simulink model "DUALportRAMinterface_v2"  (R2024a)
settings: Solver=FixedStepDiscrete  StartTime=0.0  StopTime=20  RelTol=1e-3
values from neighbouring files (symbols this model uses):
  Ts = 1/Fs    (= 7.50007500075e-06)    [new_generation_coeff.m]    (also in simon_test.m; simple_fft_test.m = 1/F; testPSD_c2d.m; testPSD_simulink.m)
undefined symbols (not defined in the file or in its folder): magnitude
libraries: hdlsllib x226, embmathops x6, simulink x1, hdlmdlgenlib x1, dsphdlxfrm2 x1
(part 2 of 5)

== system DUALportRAMinterface_v2/PL/integration_block1/FIFO_system1 ==
  data_in : Inport
  enable_output : Inport  Port=2  OutDataTypeStr=boolean
  load_fifo : Inport  Port=3  OutDataTypeStr=boolean
  Add1 : Sum  OutDataTypeStr=fixdt(0,13,0)
  Chart1 : Stateflow chart  TreatAsAtomicUnit=on
      settings: PortSchema="{\"entries\":[{\"content\":{\"sides\":[{\"content\":{\"connectorIds\":[\"In2\"]},\"type\":\"ConnectorPlacement.EquallySpacedRectSide\",\"uuid\":\"9d6f18ef-7bce-40b0-94a2-758e33355834\"},{\"content\":{\"connectorIds\":[\"Out1\"],\"side\":\"RIGHT\"},\"type\":\"ConnectorPlacement.EquallySpacedRectSide\",\"uuid\":\"7bab70ba-8111-4145-9c29-33f98ce79820\"},{\"content\":{\"side\":\"TOP\"},\"type\":\"ConnectorPlacement.EquallySpacedRectSide\",\"uuid\":\"d3288235-814f-4c71-bec2-04d07c53d63c\"},{\"content\":{\"connectorIds\":[\"In1\"],\"side\":\"BOTTOM\"},\"type\":\"ConnectorPlacement.EquallySpacedRectSide\",\"uuid\":\"018953e5-55f4-4114-8f5d-132f3f7565f7\"}]},\"type\":\"ConnectorPlacement.EquallySpacedConnector\",\"uuid\":\"70011da9-c6ae-4e69-953f-1d8cbe8c7c12\"}],\"packageUris\":[\"http://schema.mathworks.com/mf0/Connector/R2020b\"],\"version\":\"1.0\"}"
  Chart2 : Stateflow chart  TreatAsAtomicUnit=on
      settings: PortSchema="{\"entries\":[{\"content\":{\"sides\":[{\"content\":{\"connectorIds\":[\"In1\"]},\"type\":\"ConnectorPlacement.EquallySpacedRectSide\",\"uuid\":\"9d6f18ef-7bce-40b0-94a2-758e33355834\"},{\"content\":{\"connectorIds\":[\"Out1\"],\"side\":\"RIGHT\"},\"type\":\"ConnectorPlacement.EquallySpacedRectSide\",\"uuid\":\"7bab70ba-8111-4145-9c29-33f98ce79820\"},{\"content\":{\"connectorIds\":[\"In2\"],\"side\":\"TOP\"},\"type\":\"ConnectorPlacement.EquallySpacedRectSide\",\"uuid\":\"d3288235-814f-4c71-bec2-04d07c53d63c\"}]},\"type\":\"ConnectorPlacement.EquallySpacedConnector\",\"uuid\":\"70011da9-c6ae-4e69-953f-1d8cbe8c7c12\"}],\"packageUris\":[\"http://schema.mathworks.com/mf0/Connector/R2020b\"],\"version\":\"1.0\"}"
  Chart3 : Stateflow chart  TreatAsAtomicUnit=on
  Constant3 : Constant  OutDataTypeStr=fixdt(0,12,0)  SampleTime=Ts
  Constant4 : Constant  Value=0  OutDataTypeStr=fixdt(1,13,0)  SampleTime=Ts
  Delay : Delay  DelayLength=2048  InitialCondition=0  UseCircularBuffer=on
  Delay1 : Delay  DelayLength=1  InitialCondition=0  SampleTime=Ts
  Delay2 : Delay  DelayLength=1  InitialCondition=0  SampleTime=Ts
  Delay3 : Delay  DelayLength=1  InitialCondition=0
  HDL FIFO1 : hdlsllib/HDL RAMs/HDL FIFO  fifo_size=4096+2048+1  mode=Classic  ratio=1  push_msg=Warning  pop_msg=Warning  show_empty=off  show_full=on  show_num=off  LabelModeActiveChoice_Mode=Classic  rst_port=off
  Logical Operator : Logic  Operator=OR  IconShape=distinctive  AllPortsSameDT=off  OutDataTypeStr=boolean
  Logical Operator1 : Logic  IconShape=distinctive  AllPortsSameDT=off  OutDataTypeStr=boolean
  Logical Operator2 : Logic  IconShape=distinctive  AllPortsSameDT=off  OutDataTypeStr=boolean
  Logical Operator3 : Logic  Operator=XOR  IconShape=distinctive  AllPortsSameDT=off  OutDataTypeStr=boolean
  Logical Operator4 : Logic  IconShape=distinctive  AllPortsSameDT=off  OutDataTypeStr=boolean
  Logical Operator5 : Logic  Operator=XOR  IconShape=distinctive  AllPortsSameDT=off  OutDataTypeStr=boolean
  Logical Operator6 : Logic  Operator=XOR  IconShape=distinctive  AllPortsSameDT=off  OutDataTypeStr=boolean
  Switch1 : Switch  Criteria=u2 ~= 0  OutDataTypeStr=fixdt(0,13,0)  SaturateOnIntegerOverflow=off  InputSameDT=off
  Switch3 : Switch  Criteria=u2 ~= 0  SaturateOnIntegerOverflow=off  InputSameDT=off  OutDataTypeStr=Inherit: Same as first input
  tuneback : Delay  DelayLength=2048+4096+0  InitialCondition=0  UseCircularBuffer=on
  data_out : Outport
  data_valid : Outport  Port=2
  reset_fft : Outport  Port=3
  FIFO_full : Outport  Port=4
  wires:
  Delay1/1 -> Chart1/1(counter), Add1/1
  Logical Operator/1 -> HDL FIFO1/2
  HDL FIFO1/1 -> Switch3/3, data_out/1
  Switch1/1 -> Chart3/1(counter), Delay1/1
  Delay2/1 -> Logical Operator1/2
  enable_output/1 -> Chart1/2(en_out)
  Add1/1 -> Switch1/1
  Constant3/1 -> Add1/2
  HDL FIFO1/2 -> Delay3/1, Logical Operator6/1, Chart2/2(full)
  Switch3/1 -> HDL FIFO1/1
  Constant4/1 -> Switch1/3
  load_fifo/1 -> Chart2/1(load_FIFO1)
  data_in/1 -> Switch3/1
  Chart3/1(enable_pop) -> HDL FIFO1/3, Logical Operator1/1, Delay2/1, Logical Operator/2
  Chart1/1(enable_counter) -> Switch1/2
  Chart2/1(enable_push) -> Switch3/2, Logical Operator/1
  Delay/1 -> Logical Operator2/2
  Logical Operator2/1 -> Logical Operator3/1, Logical Operator5/1
  Logical Operator1/1 -> Logical Operator4/1, Logical Operator3/2, Logical Operator2/1, tuneback/1, Delay/1
  Logical Operator3/1 -> reset_fft/1
  tuneback/1 -> Logical Operator4/2
  Logical Operator4/1 -> Logical Operator5/2
  Logical Operator5/1 -> data_valid/1
  Logical Operator6/1 -> FIFO_full/1
  Delay3/1 -> Logical Operator6/2

== system DUALportRAMinterface_v2/PL/integration_block1/FIFO_system3 ==
  data_in : Inport
  enable_output : Inport  Port=2  OutDataTypeStr=boolean
  load_fifo : Inport  Port=3  OutDataTypeStr=boolean
  Add1 : Sum  OutDataTypeStr=fixdt(0,13,0)
  Chart1 : Stateflow chart  TreatAsAtomicUnit=on
      settings: PortSchema="{\"entries\":[{\"content\":{\"sides\":[{\"content\":{\"connectorIds\":[\"In2\"]},\"type\":\"ConnectorPlacement.EquallySpacedRectSide\",\"uuid\":\"9d6f18ef-7bce-40b0-94a2-758e33355834\"},{\"content\":{\"connectorIds\":[\"Out1\"],\"side\":\"RIGHT\"},\"type\":\"ConnectorPlacement.EquallySpacedRectSide\",\"uuid\":\"7bab70ba-8111-4145-9c29-33f98ce79820\"},{\"content\":{\"side\":\"TOP\"},\"type\":\"ConnectorPlacement.EquallySpacedRectSide\",\"uuid\":\"d3288235-814f-4c71-bec2-04d07c53d63c\"},{\"content\":{\"connectorIds\":[\"In1\"],\"side\":\"BOTTOM\"},\"type\":\"ConnectorPlacement.EquallySpacedRectSide\",\"uuid\":\"018953e5-55f4-4114-8f5d-132f3f7565f7\"}]},\"type\":\"ConnectorPlacement.EquallySpacedConnector\",\"uuid\":\"70011da9-c6ae-4e69-953f-1d8cbe8c7c12\"}],\"packageUris\":[\"http://schema.mathworks.com/mf0/Connector/R2020b\"],\"version\":\"1.0\"}"
  Chart2 : Stateflow chart  TreatAsAtomicUnit=on
      settings: PortSchema="{\"entries\":[{\"content\":{\"sides\":[{\"content\":{\"connectorIds\":[\"In1\"]},\"type\":\"ConnectorPlacement.EquallySpacedRectSide\",\"uuid\":\"9d6f18ef-7bce-40b0-94a2-758e33355834\"},{\"content\":{\"connectorIds\":[\"Out1\"],\"side\":\"RIGHT\"},\"type\":\"ConnectorPlacement.EquallySpacedRectSide\",\"uuid\":\"7bab70ba-8111-4145-9c29-33f98ce79820\"},{\"content\":{\"connectorIds\":[\"In2\"],\"side\":\"TOP\"},\"type\":\"ConnectorPlacement.EquallySpacedRectSide\",\"uuid\":\"d3288235-814f-4c71-bec2-04d07c53d63c\"}]},\"type\":\"ConnectorPlacement.EquallySpacedConnector\",\"uuid\":\"70011da9-c6ae-4e69-953f-1d8cbe8c7c12\"}],\"packageUris\":[\"http://schema.mathworks.com/mf0/Connector/R2020b\"],\"version\":\"1.0\"}"
  Chart3 : Stateflow chart  TreatAsAtomicUnit=on
  Constant3 : Constant  OutDataTypeStr=fixdt(0,12,0)  SampleTime=Ts
  Constant4 : Constant  Value=0  OutDataTypeStr=fixdt(1,13,0)  SampleTime=Ts
  Delay : Delay  DelayLength=2048  InitialCondition=0  UseCircularBuffer=on
  Delay1 : Delay  DelayLength=1  InitialCondition=0  SampleTime=Ts
  Delay2 : Delay  DelayLength=1  InitialCondition=0  SampleTime=Ts
  Delay3 : Delay  DelayLength=1  InitialCondition=0
  HDL FIFO1 : hdlsllib/HDL RAMs/HDL FIFO  fifo_size=4096+2048+1  mode=Classic  ratio=1  push_msg=Warning  pop_msg=Warning  show_empty=off  show_full=on  show_num=off  LabelModeActiveChoice_Mode=Classic  rst_port=off
  Logical Operator : Logic  Operator=OR  IconShape=distinctive  AllPortsSameDT=off  OutDataTypeStr=boolean
  Logical Operator1 : Logic  IconShape=distinctive  AllPortsSameDT=off  OutDataTypeStr=boolean
  Logical Operator2 : Logic  IconShape=distinctive  AllPortsSameDT=off  OutDataTypeStr=boolean
  Logical Operator3 : Logic  Operator=XOR  IconShape=distinctive  AllPortsSameDT=off  OutDataTypeStr=boolean
  Logical Operator4 : Logic  IconShape=distinctive  AllPortsSameDT=off  OutDataTypeStr=boolean
  Logical Operator5 : Logic  Operator=XOR  IconShape=distinctive  AllPortsSameDT=off  OutDataTypeStr=boolean
  Logical Operator6 : Logic  Operator=XOR  IconShape=distinctive  AllPortsSameDT=off  OutDataTypeStr=boolean
  Switch1 : Switch  Criteria=u2 ~= 0  OutDataTypeStr=fixdt(0,13,0)  SaturateOnIntegerOverflow=off  InputSameDT=off
  Switch3 : Switch  Criteria=u2 ~= 0  SaturateOnIntegerOverflow=off  InputSameDT=off  OutDataTypeStr=Inherit: Same as first input
  tuneback : Delay  DelayLength=2048+4096+0  InitialCondition=0  UseCircularBuffer=on
  data_out : Outport
  data_valid : Outport  Port=2
  reset_fft : Outport  Port=3
  FIFO_full : Outport  Port=4
  wires:
  Delay3/1 -> Logical Operator6/2
  Logical Operator6/1 -> FIFO_full/1
  Logical Operator5/1 -> data_valid/1
  Logical Operator4/1 -> Logical Operator5/2
  tuneback/1 -> Logical Operator4/2
  Logical Operator3/1 -> reset_fft/1
  Logical Operator1/1 -> Delay/1, tuneback/1, Logical Operator2/1, Logical Operator3/2, Logical Operator4/1
  Logical Operator2/1 -> Logical Operator5/1, Logical Operator3/1
  Delay/1 -> Logical Operator2/2
  Chart2/1(enable_push) -> Logical Operator/1, Switch3/2
  Chart1/1(enable_counter) -> Switch1/2
  Chart3/1(enable_pop) -> Logical Operator/2, Delay2/1, Logical Operator1/1, HDL FIFO1/3
  data_in/1 -> Switch3/1
  load_fifo/1 -> Chart2/1(load_FIFO1)
  Constant4/1 -> Switch1/3
  Switch3/1 -> HDL FIFO1/1
  HDL FIFO1/2 -> Chart2/2(full), Logical Operator6/1, Delay3/1
  Constant3/1 -> Add1/2
  Add1/1 -> Switch1/1
  enable_output/1 -> Chart1/2(en_out)
  Delay2/1 -> Logical Operator1/2
  Switch1/1 -> Delay1/1, Chart3/1(counter)
  HDL FIFO1/1 -> data_out/1, Switch3/3
  Logical Operator/1 -> HDL FIFO1/2
  Delay1/1 -> Add1/1, Chart1/1(counter)

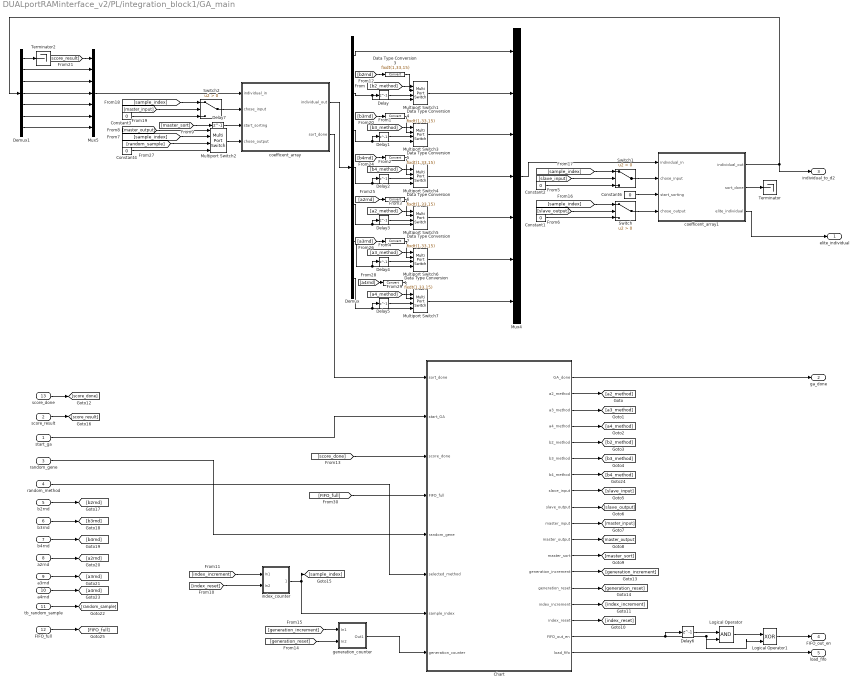
== system DUALportRAMinterface_v2/PL/integration_block1/GA_main ==
  start_ga : Inport
  score_result : Inport  Port=2
  random_gene : Inport  Port=3
  random_method : Inport  Port=4
  b2rnd : Inport  Port=5
  b3rnd : Inport  Port=6
  b4rnd : Inport  Port=7
  a2rnd : Inport  Port=8
  a3rnd : Inport  Port=9
  a4rnd : Inport  Port=10
  tb_random_sample : Inport  Port=11
  FIFO_full : Inport  Port=12
  score_done : Inport  Port=13
  Chart : Stateflow chart  TreatAsAtomicUnit=on
      settings: PortSchema="{\"entries\":[{\"content\":{\"sides\":[{\"content\":{\"connectorIds\":[\"In1\",\"In2\",\"In3\",\"In4\",\"In5\",\"In6\",\"In7\",\"In8\"]},\"type\":\"ConnectorPlacement.EquallySpacedRectSide\",\"uuid\":\"62d80992-ebbf-487b-a33b-520d46b16df9\"},{\"content\":{\"connectorIds\":[\"Out1\",\"Out4\",\"Out5\",\"Out6\",\"Out8\",\"Out9\",\"Out7\",\"Out10\",\"Out11\",\"Out12\",\"Out15\",\"Out16\",\"Out13\",\"Out14\",\"Out3\",\"Out2\",\"Out17\",\"Out18\"],\"side\":\"RIGHT\"},\"type\":\"ConnectorPlacement.EquallySpacedRectSide\",\"uuid\":\"bfd840c0-5c4c-4a80-a2e3-fe311b40edf5\"},{\"content\":{\"side\":\"TOP\"},\"type\":\"ConnectorPlacement.EquallySpacedRectSide\",\"uuid\":\"4ac6e66e-dbf9-46cb-9f74-339923e0521f\"},{\"content\":{\"side\":\"BOTTOM\"},\"type\":\"ConnectorPlacement.EquallySpacedRectSide\",\"uuid\":\"c9defcd3-49e4-4e79-8497-0d4d1ccc3a89\"}]},\"type\":\"ConnectorPlacement.EquallySpacedConnector\",\"uuid\":\"f0f6ce29-0824-409a-b95e-7d534cdcf216\"}],\"packageUris\":[\"http://schema.mathworks.com/mf0/Connector/R2020b\"],\"version\":\"1.0\"}"
  Constant{1..4} (4 alike) : Constant  Value=0  OutDataTypeStr=fixdt(0,4,0)  SampleTime=Ts
  Constant6 : Constant  Value=0  OutDataTypeStr=boolean  SampleTime=Ts
  Data Type Conversion{1,3..7} (6 alike) : DataTypeConversion  OutDataTypeStr=fixdt(1,33,15)  SaturateOnIntegerOverflow=off  RndMeth=Floor
  Delay{,1..6} (7 alike) : Delay  DelayLength=1  InitialCondition=0
  Delay7 : Delay  DelayLength=1  SampleTime=Ts
  Demux : Demux  Outputs=7
  Demux1 : Demux  Outputs=7
  Logical Operator : Logic  IconShape=distinctive  AllPortsSameDT=off  OutDataTypeStr=boolean
  Logical Operator1 : Logic  Operator=XOR  IconShape=distinctive  AllPortsSameDT=off  OutDataTypeStr=boolean
  Multiport Switch{1,3..7} (6 alike) : MultiPortSwitch  DiagnosticForDefault=None  OutDataTypeStr=Inherit: Same as first data input  SaturateOnIntegerOverflow=off  InputSameDT=off
  Multiport Switch2 : MultiPortSwitch  DiagnosticForDefault=None  SaturateOnIntegerOverflow=off  InputSameDT=off
  Mux4 : Mux  Inputs=7
  Mux5 : Mux  Inputs=7
  Switch : Switch  Criteria=u2 > Threshold  SaturateOnIntegerOverflow=off  InputSameDT=off
  Switch1 : Switch  Criteria=u2 > Threshold  SaturateOnIntegerOverflow=off  InputSameDT=off
  Switch2 : Switch  Criteria=u2 > Threshold  OutDataTypeStr=fixdt(0,4,0)  SaturateOnIntegerOverflow=off  InputSameDT=off
  Terminator : Terminator
  Terminator2 : Terminator
  coefficent_array : Subsystem
  coefficent_array1 : Subsystem
  generation_counter : Subsystem
  index_counter : Subsystem
  elite_individual : Outport  OutDataTypeStr=fixdt(1,33,15)
  ga_done : Outport  Port=2  OutDataTypeStr=boolean
  individual_to_d2 : Outport  Port=3
  FIFO_out_en : Outport  Port=4
  load_fifo : Outport  Port=5
  wires:
  Demux/2 -> Multiport Switch1/4, Delay/1
  Chart/5(a3_method) -> [a3_method]
  coefficent_array1/1(individual_out) -> individual_to_d2/1, Demux1/1
  index_counter/1(index_counter) -> [sample_index], Chart/7(sample_index)
  Chart/13(generation_increment) -> [generation_increment]
  [a3rnd] -> Data Type Conversion7/1
  Delay2/1 -> Multiport Switch4/3
  [b4_method] -> Multiport Switch4/1
  Demux/1 -> Mux4/1
  Delay7/1 -> coefficent_array/3(start_sorting)
  Delay4/1 -> Multiport Switch6/3
  Demux1/4 -> Mux5/4
  Multiport Switch3/1 -> Mux4/3
  Demux/5 -> Multiport Switch5/4, Delay3/1
  Chart/4(a2_method) -> [a2_method]
  generation_counter/1(Out1) -> Chart/8(generation_counter)
  Delay3/1 -> Multiport Switch5/3
  coefficent_array/1(individual_out) -> Demux/1
  Data Type Conversion5/1 -> Multiport Switch4/2
  [b4rnd] -> Data Type Conversion5/1
  Data Type Conversion4/1 -> Multiport Switch3/2
  [b2rnd] -> Data Type Conversion3/1
  [slave_output] -> Switch/2
  Multiport Switch2/1 -> coefficent_array/4(chose_output)
  Demux/6 -> Multiport Switch6/4, Delay4/1
  Multiport Switch6/1 -> Mux4/6
  Data Type Conversion7/1 -> Multiport Switch6/2
  Mux5/1 -> coefficent_array/1(individual_in)
  coefficent_array/2(sort_done) -> Chart/1(sort_done)
  [b3_method] -> Multiport Switch3/1
  [a2rnd] -> Data Type Conversion6/1
  Chart/6(a4_method) -> [a4_method]
  [b3rnd] -> Data Type Conversion4/1
  Mux4/1 -> coefficent_array1/1(individual_in)
  Multiport Switch5/1 -> Mux4/5
  [a2_method] -> Multiport Switch5/1
  [master_output] -> Multiport Switch2/1
  Switch1/1 -> coefficent_array1/2(chose_input)
  Chart/11(slave_output) -> [slave_output]
  [b2_method] -> Multiport Switch1/1
  [master_sort] -> Delay7/1
  [index_reset] -> index_counter/2(In2)
  Delay/1 -> Multiport Switch1/3
  Chart/8(b2_method) -> [b2_method]
  Demux1/3 -> Mux5/3
  Demux/4 -> Multiport Switch4/4, Delay2/1
  [generation_reset] -> generation_counter/2(In2)
  Data Type Conversion6/1 -> Multiport Switch5/2
  [sample_index] -> Switch/1
  Switch2/1 -> coefficent_array/2(chose_input)
  Chart/9(b3_method) -> [b3_method]
  Chart/15(master_output) -> [master_output]
  Demux/3 -> Multiport Switch3/4, Delay1/1
  Chart/10(slave_input) -> [slave_input]
  Chart/2(index_reset) -> [index_reset]
  Demux1/1 -> Terminator2/1
  Demux1/5 -> Mux5/5
  [score_done] -> Chart/3(score_done)
  Chart/3(index_increment) -> [index_increment]
  Constant1/1 -> Switch/3
  Demux1/6 -> Mux5/6
  [sample_index] -> Switch1/1
  Chart/16(master_sort) -> [master_sort]
  Constant3/1 -> Switch2/3
  Switch/1 -> coefficent_array1/4(chose_output)
  [generation_increment] -> generation_counter/1(In1)
  Chart/12(master_input) -> [master_input]
  Constant4/1 -> Multiport Switch2/4
  [a3_method] -> Multiport Switch6/1
  Constant6/1 -> coefficent_array1/3(start_sorting)
  [sample_index] -> Multiport Switch2/2
  Multiport Switch1/1 -> Mux4/2
  Demux1/2 -> Mux5/2
  Chart/14(generation_reset) -> [generation_reset]
  Constant2/1 -> Switch1/3
  [index_increment] -> index_counter/1(In1)
  [sample_index] -> Switch2/1
  [master_input] -> Switch2/2
  Delay1/1 -> Multiport Switch3/3
  [slave_input] -> Switch1/2
  Data Type Conversion3/1 -> Multiport Switch1/2
  Chart/1(GA_done) -> ga_done/1
  Multiport Switch4/1 -> Mux4/4
  coefficent_array1/2(sort_done) -> Terminator/1
  [score_result] -> Mux5/1
  start_ga/1 -> Chart/2(start_GA)
  score_done/1 -> [score_done]
  score_result/1 -> [score_result]
  random_gene/1 -> Chart/5(random_gene)
  random_method/1 -> Chart/6(selected_method)
  b2rnd/1 -> [b2rnd]
  b3rnd/1 -> [b3rnd]
  b4rnd/1 -> [b4rnd]
  a2rnd/1 -> [a2rnd]
  a3rnd/1 -> [a3rnd]
  [random_sample] -> Multiport Switch2/3
  tb_random_sample/1 -> [random_sample]
  Demux1/7 -> Mux5/7
  [a4_method] -> Multiport Switch7/1
  Data Type Conversion1/1 -> Multiport Switch7/2
  Multiport Switch7/1 -> Mux4/7
  Demux/7 -> Delay5/1, Multiport Switch7/4
  Delay5/1 -> Multiport Switch7/3
  [a4rnd] -> Data Type Conversion1/1
  a4rnd/1 -> [a4rnd]
  Chart/7(b4_method) -> [b4_method]
  FIFO_full/1 -> [FIFO_full]
  [FIFO_full] -> Chart/4(FIFO_full)
  Chart/18(load_fifo) -> load_fifo/1
  Delay6/1 -> Logical Operator/1
  Chart/17(FIFO_out_en) -> Delay6/1, Logical Operator1/2, Logical Operator/2
  Logical Operator/1 -> Logical Operator1/1
  Logical Operator1/1 -> FIFO_out_en/1
  coefficent_array1/3(elite_individual) -> elite_individual/1

== system DUALportRAMinterface_v2/PL/integration_block1/Subsystem ==
  enable : Inport
  16bLFSR : Subsystem
  16bLFSR1 : Subsystem
  Terminator13 : Terminator
  Terminator14 : Terminator
  a2_random : Subsystem
  a3_random : Subsystem
  a4_random : Subsystem
  b2_random : Subsystem
  b3_random : Subsystem
  b4_random : Subsystem
  concat : hdlsllib/Logic and Bit Operations/Bit Concat  numInputs=16
  random_gene : Subsystem
  random_method : Subsystem
  random_sample : Subsystem
  random_gene_out : Outport
  random_method_out : Outport  Port=2
  b2_random_out : Outport  Port=3
  b3_random_out : Outport  Port=4
  b4_random_out : Outport  Port=5
  a2_random_out : Outport  Port=6
  a3_random_out : Outport  Port=7
  a4_random_out : Outport  Port=8
  random_sample_out : Outport  Port=9
  wires:
  16bLFSR/11(y10) -> concat/11
  16bLFSR1/10(y9) -> random_gene/1(u1)
  16bLFSR/5(y4) -> concat/5
  16bLFSR/10(y9) -> concat/10
  enable/1 -> 16bLFSR1/1(In1), 16bLFSR/1(In1)
  16bLFSR1/9(y8) -> random_method/2(u2)
  16bLFSR1/12(y11) -> random_gene/3(In3)
  concat/1 -> a3_random/1(In1), a2_random/1(In1), b3_random/1(In1), b2_random/1(In1), b4_random/1(In1), a4_random/1(In1)
  16bLFSR1/13(y12) -> b3_random/2(In2)
  a4_random/1(Out1) -> a4_random_out/1
  16bLFSR/1(y_port) -> concat/1
  16bLFSR/6(y5) -> concat/6
  16bLFSR1/11(y10) -> random_gene/2(u2)
  random_gene/1(Out1) -> random_gene_out/1
  16bLFSR/14(y13) -> concat/14
  16bLFSR1/14(y13) -> random_gene/4(In4)
  16bLFSR/12(y11) -> concat/12
  a3_random/1(Out1) -> a3_random_out/1
  16bLFSR1/3(y2) -> a4_random/2(In2)
  16bLFSR/4(y3) -> concat/4
  16bLFSR/13(y12) -> concat/13
  16bLFSR/16(y15) -> concat/16
  random_method/1(Out1) -> random_method_out/1
  16bLFSR1/6(y5) -> random_sample/1(u1)
  16bLFSR/2(y1) -> concat/2
  16bLFSR/3(y2) -> concat/3
  16bLFSR1/8(y7) -> random_method/1(u1)
  b2_random/1(Out1) -> b2_random_out/1
  16bLFSR/15(y14) -> concat/15
  16bLFSR1/2(y1) -> a3_random/2(In2)
  16bLFSR1/7(y6) -> random_sample/2(u2)
  16bLFSR1/1(y_port) -> a2_random/2(In2)
  16bLFSR1/5(y4) -> b4_random/2(In2)
  16bLFSR1/15(y14) -> Terminator13/1
  16bLFSR/8(y7) -> concat/8
  a2_random/1(Out1) -> a2_random_out/1
  random_sample/1(Out1) -> random_sample_out/1
  16bLFSR/9(y8) -> concat/9
  b4_random/1(Out1) -> b4_random_out/1
  16bLFSR/7(y6) -> concat/7
  16bLFSR1/16(y15) -> Terminator14/1
  16bLFSR1/4(y3) -> b2_random/2(In2)
  b3_random/1(Out1) -> b3_random_out/1

== system DUALportRAMinterface_v2/PL/integration_block1/accumulator_scorer ==
  data_in : Inport
  valid_fft : Inport  Port=2
  64bitmsb_finder : Subsystem
  Add : Sum  OutDataTypeStr=fixdt(1,64,32)  AccumDataTypeStr=fixdt(1,64,32)  SaturateOnIntegerOverflow=on
  Add2 : Sum  AccumDataTypeStr=fixdt(1,64,32)  SaturateOnIntegerOverflow=on  OutDataTypeStr=Inherit: Same as first input
  Complex to Real-Imag : ComplexToRealImag
  Constant1 : Constant  Value=0  OutDataTypeStr=fixdt(1,26,12)  SampleTime=Ts
  Constant19 : Constant  Value=0  OutDataTypeStr=fixdt(1,26,12)  SampleTime=Ts
  Constant20 : Constant  Value=0  OutDataTypeStr=fixdt(1,64,32)  SampleTime=Ts
  Data Type Conversion : DataTypeConversion  OutDataTypeStr=fixdt(1,64,32)  SaturateOnIntegerOverflow=off  RndMeth=Floor
  Data Type Conversion1 : DataTypeConversion  OutDataTypeStr=fixdt(1,64,32)  SaturateOnIntegerOverflow=off  RndMeth=Floor
  Data Type Conversion2 : DataTypeConversion  OutDataTypeStr=fixdt(1,33,15)  SaturateOnIntegerOverflow=off  RndMeth=Floor
  Delay : Delay  DelayLength=1  InitialCondition=0  SampleTime=Ts
  Delay1 : Delay  DelayLength=63  InitialCondition=0
  Delay2 : Delay  DelayLength=1  InitialCondition=0
  Delay3 : Delay  DelayLength=4096-64  InitialCondition=0  UseCircularBuffer=on
  Logical Operator1 : Logic  IconShape=distinctive  AllPortsSameDT=off  OutDataTypeStr=boolean
  Logical Operator2 : Logic  IconShape=distinctive  AllPortsSameDT=off  OutDataTypeStr=boolean
  Magnitude Square1 : Math  Operator=magnitude^2  SignedPower=on  OutputSignalType=real  RndMeth=Zero
  Magnitude Square2 : Math  Operator=magnitude^2  SignedPower=on  OutputSignalType=real  RndMeth=Zero
  Real-Imag to Complex : RealImagToComplex
  Switch : Switch  Criteria=u2 > Threshold  SaturateOnIntegerOverflow=off  InputSameDT=off  OutDataTypeStr=Inherit: Same as first input
  Switch8 : Switch  Criteria=u2 > Threshold  OutDataTypeStr=fixdt(1,64,32)  InputSameDT=off
  individual_score : Outport
  individual_score_valid : Outport  Port=2
  wires:
  Real-Imag to Complex/1 -> Switch/3
  Switch8/1 -> Add/2
  Switch/1 -> Complex to Real-Imag/1
  Delay/1 -> Data Type Conversion2/1, Switch8/1
  [reset_lol] -> Switch8/2
  Add/1 -> Delay/1
  Constant20/1 -> Switch8/3
  Complex to Real-Imag/2 -> Data Type Conversion1/1
  Complex to Real-Imag/1 -> Data Type Conversion/1
  Magnitude Square1/1 -> Add2/1
  Add2/1 -> 64bitmsb_finder/1(u_port)
  Magnitude Square2/1 -> Add2/2
  Logical Operator1/1 -> [reset_lol], Logical Operator2/2, Switch/2, Delay1/1
  data_in/1 -> Switch/1
  Constant1/1 -> Real-Imag to Complex/2
  Constant19/1 -> Real-Imag to Complex/1
  Delay1/1 -> Logical Operator2/1
  Logical Operator2/1 -> Delay2/1
  Delay2/1 -> individual_score_valid/1
  valid_fft/1 -> Delay3/1, Logical Operator1/1
  Delay3/1 -> Logical Operator1/2
  64bitmsb_finder/1(out1) -> Add/1
  Data Type Conversion/1 -> Magnitude Square1/1
  Data Type Conversion1/1 -> Magnitude Square2/1
  Data Type Conversion2/1 -> individual_score/1

== system DUALportRAMinterface_v2/PL/integration_block1/D2/individual1 ==
  reg_in : Inport
  reg_in1 : Inport  Port=2
  reg_in2 : Inport  Port=3
  reg_in3 : Inport  Port=4
  reg_in4 : Inport  Port=5
  reg_in5 : Inport  Port=6
  reg_in6 : Inport  Port=7
  enable : Inport  Port=8
  Subsystem : Subsystem
  Subsystem1 : Subsystem
  Subsystem2 : Subsystem
  Subsystem3 : Subsystem
  Subsystem4 : Subsystem
  Subsystem5 : Subsystem
  Subsystem6 : Subsystem
  score : Outport
  a2 : Outport  Port=2
  a3 : Outport  Port=3
  a4 : Outport  Port=4
  b2 : Outport  Port=5
  b3 : Outport  Port=6
  b4 : Outport  Port=7
  wires:
  enable/1 -> Subsystem3/2(enable), Subsystem4/2(enable), Subsystem5/2(enable), Subsystem6/2(enable), Subsystem2/2(enable), Subsystem1/2(enable), Subsystem/2(enable)
  Subsystem2/1(reg_out) -> a3/1
  Subsystem4/1(reg_out) -> b2/1
  Subsystem3/1(reg_out) -> a4/1
  Subsystem1/1(reg_out) -> a2/1
  reg_in/1 -> Subsystem/1(reg_in)
  Subsystem/1(reg_out) -> score/1
  reg_in1/1 -> Subsystem1/1(reg_in)
  reg_in2/1 -> Subsystem2/1(reg_in)
  reg_in3/1 -> Subsystem3/1(reg_in)
  Subsystem5/1(reg_out) -> b3/1
  reg_in4/1 -> Subsystem4/1(reg_in)
  reg_in5/1 -> Subsystem5/1(reg_in)
  Subsystem6/1(reg_out) -> b4/1
  reg_in6/1 -> Subsystem6/1(reg_in)

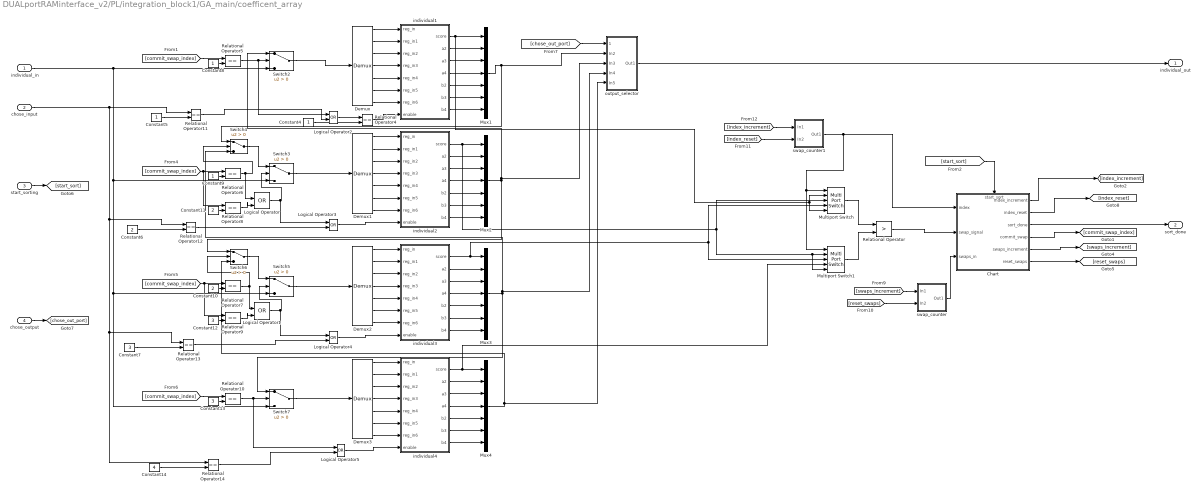
== system DUALportRAMinterface_v2/PL/integration_block1/GA_main/coefficent_array ==
  individual_in : Inport
  chose_input : Inport  Port=2
  start_sorting : Inport  Port=3
  chose_output : Inport  Port=4
  Chart : Stateflow chart  TreatAsAtomicUnit=on
      settings: PortSchema="{\"entries\":[{\"content\":{\"sides\":[{\"content\":{\"connectorIds\":[\"In1\",\"In4\",\"In3\"]},\"type\":\"ConnectorPlacement.EquallySpacedRectSide\",\"uuid\":\"bd2dafac-a5a9-4836-b8bd-cefb36fb6626\"},{\"content\":{\"connectorIds\":[\"Out1\",\"Out2\",\"Out3\",\"Out4\",\"Out5\",\"Out6\"],\"side\":\"RIGHT\"},\"type\":\"ConnectorPlacement.EquallySpacedRectSide\",\"uuid\":\"b2eb894e-8d56-4038-acbe-51c43d919a15\"},{\"content\":{\"connectorIds\":[\"In2\"],\"side\":\"TOP\"},\"type\":\"ConnectorPlacement.EquallySpacedRectSide\",\"uuid\":\"645ecb99-1eca-4a2d-8e44-d34ac75e3d1a\"}]},\"type\":\"ConnectorPlacement.EquallySpacedConnector\",\"uuid\":\"63f53eab-c5ec-482c-b992-d953653b0c27\"}],\"packageUris\":[\"http://schema.mathworks.com/mf0/Connector/R2020b\"],\"version\":\"1.0\"}"
  Constant10 : Constant  Value=2  OutDataTypeStr=fixdt(0,4,0)  SampleTime=Ts
  Constant11 : Constant  Value=2  OutDataTypeStr=fixdt(0,4,0)  SampleTime=Ts
  Constant12 : Constant  Value=3  OutDataTypeStr=fixdt(0,4,0)  SampleTime=Ts
  Constant13 : Constant  Value=3  OutDataTypeStr=fixdt(0,4,0)  SampleTime=Ts
  Constant14 : Constant  Value=4  OutDataTypeStr=fixdt(0,4,0)  SampleTime=Ts
  Constant{4..5,8..9} (4 alike) : Constant  OutDataTypeStr=fixdt(0,4,0)  SampleTime=Ts
  Constant6 : Constant  Value=2  OutDataTypeStr=fixdt(0,4,0)  SampleTime=Ts
  Constant7 : Constant  Value=3  OutDataTypeStr=fixdt(0,4,0)  SampleTime=Ts
  Demux{,1..3} (4 alike) : Demux  Outputs=7
  Logical Operator{,1..5} (6 alike) : Logic  Operator=OR  IconShape=distinctive  AllPortsSameDT=off  OutDataTypeStr=boolean
  Multiport Switch : MultiPortSwitch  DataPortForDefault=Additional data port  DiagnosticForDefault=None  SaturateOnIntegerOverflow=off  InputSameDT=off
  Multiport Switch1 : MultiPortSwitch  DataPortForDefault=Additional data port  DiagnosticForDefault=None  SaturateOnIntegerOverflow=off  InputSameDT=off
  Mux{1..4} (4 alike) : Mux  Inputs=7
  Relational Operator : RelationalOperator  Operator=>  OutDataTypeStr=boolean  InputSameDT=off
  Relational Operator{4..14} (11 alike) : RelationalOperator  Operator===  OutDataTypeStr=boolean  RndMeth=Simplest  InputSameDT=off
  Switch{2..7} (6 alike) : Switch  Criteria=u2 > Threshold  SaturateOnIntegerOverflow=off  InputSameDT=off
  individual1 : Subsystem
  individual2 : Subsystem
  individual3 : Subsystem
  individual4 : Subsystem
  output_selector : Subsystem
  swap_counter : Subsystem
  swap_counter1 : Subsystem
  individual_out : Outport
  sort_done : Outport  Port=2
  wires:
  Logical Operator1/1 -> Logical Operator4/1, Switch5/2
  Constant9/1 -> Relational Operator6/2
  Chart/5(swaps_increment) -> [swaps_increment]
  swap_counter1/1(Out1) -> Multiport Switch1/1, Multiport Switch/1, Chart/1(index)
  Switch4/1 -> Switch3/1
  individual1/1(score) -> Mux1/1, Multiport Switch/5, Multiport Switch/2
  Demux/1 -> individual1/1(reg_in)
  Mux3/1 -> output_selector/4(In4), Switch4/3, Switch7/1
  Relational Operator10/1 -> Logical Operator5/1, Switch7/2
  [reset_swaps] -> swap_counter/2(In2)
  swap_counter/1(Out1) -> Chart/3(swaps_in)
  individual1/3(a3) -> Mux1/3
  Relational Operator5/1 -> Logical Operator2/1, Switch2/2
  [swaps_increment] -> swap_counter/1(In1)
  [commit_swap_index] -> Relational Operator5/1
  Mux1/1 -> Switch4/1, output_selector/2(In2)
  Chart/6(reset_swaps) -> [reset_swaps]
  Relational Operator8/1 -> Logical Operator/2
  [commit_swap_index] -> Relational Operator8/1, Relational Operator6/1
  [commit_swap_index] -> Relational Operator9/1, Relational Operator7/1
  Logical Operator3/1 -> individual2/8(enable)
  Logical Operator5/1 -> individual4/8(enable)
  Multiport Switch/1 -> Relational Operator/1
  Constant11/1 -> Relational Operator8/2
  start_sorting/1 -> [start_sort]
  Chart/4(commit_swap) -> [commit_swap_index]
  Logical Operator/1 -> Logical Operator3/1, Switch3/2
  Demux/5 -> individual1/5(reg_in4)
  individual_in/1 -> Switch7/3, Switch5/3, Switch3/3, Switch2/3
  Switch3/1 -> Demux1/1
  individual4/1(score) -> Multiport Switch1/4, Mux4/1
  Relational Operator6/1 -> Logical Operator/1, Switch4/2
  Constant4/1 -> Relational Operator4/2
  Constant13/1 -> Relational Operator10/2
  Constant12/1 -> Relational Operator9/2
  [commit_swap_index] -> Relational Operator10/1
  Switch6/1 -> Switch5/1
  output_selector/1(Out1) -> individual_out/1
  individual2/1(score) -> Mux2/1, Multiport Switch/3, Multiport Switch1/5, Multiport Switch1/2
  [chose_out_port] -> output_selector/1(chose_port)
  Demux/6 -> individual1/6(reg_in5)
  chose_input/1 -> Relational Operator14/1, Relational Operator13/1, Relational Operator12/1, Relational Operator11/1
  Relational Operator/1 -> Chart/4(swap_signal)
  Logical Operator4/1 -> individual3/8(enable)
  Demux/3 -> individual1/3(reg_in2)
  Mux2/1 -> output_selector/3(In3), Switch2/1, Switch6/1
  individual3/1(score) -> Mux3/1, Multiport Switch1/3, Multiport Switch/4
  Constant8/1 -> Relational Operator5/2
  Switch7/1 -> Demux3/1
  Chart/1(index_increment) -> [index_increment]
  Switch5/1 -> Demux2/1
  individual2/2(a2) -> Mux2/2
  Relational Operator7/1 -> Logical Operator1/1, Switch6/2
  Multiport Switch1/1 -> Relational Operator/2
  Switch2/1 -> Demux/1
  Relational Operator9/1 -> Logical Operator1/2
  Constant10/1 -> Relational Operator7/2
  Logical Operator2/1 -> Relational Operator4/1
  individual1/5(b2) -> Mux1/5
  Demux/2 -> individual1/2(reg_in1)
  individual1/6(b3) -> Mux1/6
  Relational Operator4/1 -> individual1/8(enable)
  individual1/2(a2) -> Mux1/2
  Demux/4 -> individual1/4(reg_in3)
  individual1/4(a4) -> Mux1/4
  individual2/3(a3) -> Mux2/3
  [start_sort] -> Chart/2(start_sort)
  Chart/3(sort_done) -> sort_done/1
  chose_output/1 -> [chose_out_port]
  Constant5/1 -> Relational Operator11/2
  Relational Operator11/1 -> Logical Operator2/2
  Constant6/1 -> Relational Operator12/2
  Relational Operator12/1 -> Logical Operator3/2
  Constant7/1 -> Relational Operator13/2
  Relational Operator13/1 -> Logical Operator4/2
  Relational Operator14/1 -> Logical Operator5/2
  Constant14/1 -> Relational Operator14/2
  [index_increment] -> swap_counter1/1(In1)
  [index_reset] -> swap_counter1/2(In2)
  Chart/2(index_reset) -> [index_reset]
  Mux4/1 -> Switch6/3, output_selector/5(In5)
  Demux/7 -> individual1/7(reg_in6)
  individual1/7(b4) -> Mux1/7
  individual2/4(a4) -> Mux2/4
  individual2/5(b2) -> Mux2/5
  individual2/6(b3) -> Mux2/6
  individual2/7(b4) -> Mux2/7
  Demux1/7 -> individual2/7(reg_in6)
  Demux1/1 -> individual2/1(reg_in)
  Demux1/2 -> individual2/2(reg_in1)
  Demux1/3 -> individual2/3(reg_in2)
  Demux1/4 -> individual2/4(reg_in3)
  Demux1/5 -> individual2/5(reg_in4)
  Demux1/6 -> individual2/6(reg_in5)
  Demux2/1 -> individual3/1(reg_in)
  Demux2/2 -> individual3/2(reg_in1)
  Demux2/3 -> individual3/3(reg_in2)
  Demux2/4 -> individual3/4(reg_in3)
  Demux2/5 -> individual3/5(reg_in4)
  Demux2/6 -> individual3/6(reg_in5)
  Demux2/7 -> individual3/7(reg_in6)
  individual3/2(a2) -> Mux3/2
  individual3/3(a3) -> Mux3/3
  individual3/4(a4) -> Mux3/4
  individual3/5(b2) -> Mux3/5
  individual3/6(b3) -> Mux3/6
  individual3/7(b4) -> Mux3/7
  Demux3/1 -> individual4/1(reg_in)
  Demux3/2 -> individual4/2(reg_in1)
  Demux3/3 -> individual4/3(reg_in2)
  Demux3/4 -> individual4/4(reg_in3)
  Demux3/5 -> individual4/5(reg_in4)
  Demux3/6 -> individual4/6(reg_in5)
  Demux3/7 -> individual4/7(reg_in6)
  individual4/2(a2) -> Mux4/2
  individual4/3(a3) -> Mux4/3
  individual4/4(a4) -> Mux4/4
  individual4/5(b2) -> Mux4/5
  individual4/6(b3) -> Mux4/6
  individual4/7(b4) -> Mux4/7

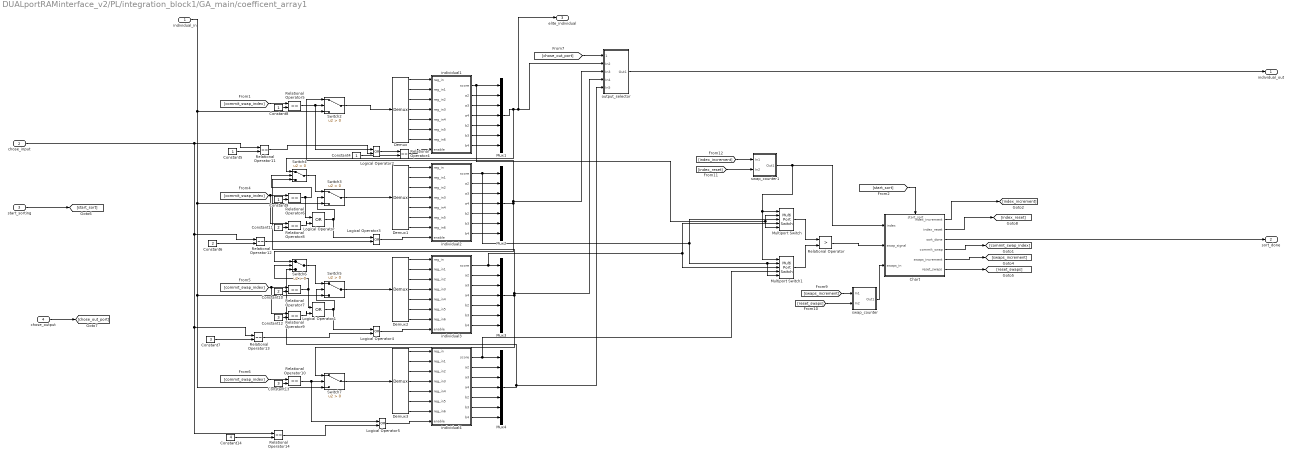
== system DUALportRAMinterface_v2/PL/integration_block1/GA_main/coefficent_array1 ==
  individual_in : Inport
  chose_input : Inport  Port=2
  start_sorting : Inport  Port=3
  chose_output : Inport  Port=4
  Chart : Stateflow chart  TreatAsAtomicUnit=on
      settings: PortSchema="{\"entries\":[{\"content\":{\"sides\":[{\"content\":{\"connectorIds\":[\"In1\",\"In4\",\"In3\"]},\"type\":\"ConnectorPlacement.EquallySpacedRectSide\",\"uuid\":\"bd2dafac-a5a9-4836-b8bd-cefb36fb6626\"},{\"content\":{\"connectorIds\":[\"Out1\",\"Out2\",\"Out3\",\"Out4\",\"Out5\",\"Out6\"],\"side\":\"RIGHT\"},\"type\":\"ConnectorPlacement.EquallySpacedRectSide\",\"uuid\":\"b2eb894e-8d56-4038-acbe-51c43d919a15\"},{\"content\":{\"connectorIds\":[\"In2\"],\"side\":\"TOP\"},\"type\":\"ConnectorPlacement.EquallySpacedRectSide\",\"uuid\":\"645ecb99-1eca-4a2d-8e44-d34ac75e3d1a\"}]},\"type\":\"ConnectorPlacement.EquallySpacedConnector\",\"uuid\":\"63f53eab-c5ec-482c-b992-d953653b0c27\"}],\"packageUris\":[\"http://schema.mathworks.com/mf0/Connector/R2020b\"],\"version\":\"1.0\"}"
  Constant10 : Constant  Value=2  OutDataTypeStr=fixdt(0,4,0)  SampleTime=Ts
  Constant11 : Constant  Value=2  OutDataTypeStr=fixdt(0,4,0)  SampleTime=Ts
  Constant12 : Constant  Value=3  OutDataTypeStr=fixdt(0,4,0)  SampleTime=Ts
  Constant13 : Constant  Value=3  OutDataTypeStr=fixdt(0,4,0)  SampleTime=Ts
  Constant14 : Constant  Value=4  OutDataTypeStr=fixdt(0,4,0)  SampleTime=Ts
  Constant{4..5,8..9} (4 alike) : Constant  OutDataTypeStr=fixdt(0,4,0)  SampleTime=Ts
  Constant6 : Constant  Value=2  OutDataTypeStr=fixdt(0,4,0)  SampleTime=Ts
  Constant7 : Constant  Value=3  OutDataTypeStr=fixdt(0,4,0)  SampleTime=Ts
  Demux{,1..3} (4 alike) : Demux  Outputs=7
  Logical Operator{,1..5} (6 alike) : Logic  Operator=OR  IconShape=distinctive  AllPortsSameDT=off  OutDataTypeStr=boolean
  Multiport Switch : MultiPortSwitch  DataPortForDefault=Additional data port  DiagnosticForDefault=None  SaturateOnIntegerOverflow=off  InputSameDT=off
  Multiport Switch1 : MultiPortSwitch  DataPortForDefault=Additional data port  DiagnosticForDefault=None  SaturateOnIntegerOverflow=off  InputSameDT=off
  Mux{1..4} (4 alike) : Mux  Inputs=7
  Relational Operator : RelationalOperator  Operator=>  OutDataTypeStr=boolean  InputSameDT=off
  Relational Operator{4..14} (11 alike) : RelationalOperator  Operator===  OutDataTypeStr=boolean  RndMeth=Simplest  InputSameDT=off
  Switch2 : Switch  Criteria=u2 > Threshold  SaturateOnIntegerOverflow=off  InputSameDT=off  OutDataTypeStr=Inherit: Same as first input
  Switch{3..7} (5 alike) : Switch  Criteria=u2 > Threshold  SaturateOnIntegerOverflow=off  InputSameDT=off
  individual1 : Subsystem
  individual2 : Subsystem
  individual3 : Subsystem
  individual4 : Subsystem
  output_selector : Subsystem
  swap_counter : Subsystem
  swap_counter1 : Subsystem
  individual_out : Outport
  sort_done : Outport  Port=2
  elite_individual : Outport  Port=3
  wires:
  individual4/7(b4) -> Mux4/7
  individual4/6(b3) -> Mux4/6
  individual4/5(b2) -> Mux4/5
  individual4/4(a4) -> Mux4/4
  individual4/3(a3) -> Mux4/3
  individual4/2(a2) -> Mux4/2
  Demux3/7 -> individual4/7(reg_in6)
  Demux3/6 -> individual4/6(reg_in5)
  Demux3/5 -> individual4/5(reg_in4)
  Demux3/4 -> individual4/4(reg_in3)
  Demux3/3 -> individual4/3(reg_in2)
  Demux3/2 -> individual4/2(reg_in1)
  Demux3/1 -> individual4/1(reg_in)
  individual3/7(b4) -> Mux3/7
  individual3/6(b3) -> Mux3/6
  individual3/5(b2) -> Mux3/5
  individual3/4(a4) -> Mux3/4
  individual3/3(a3) -> Mux3/3
  individual3/2(a2) -> Mux3/2
  Demux2/7 -> individual3/7(reg_in6)
  Demux2/6 -> individual3/6(reg_in5)
  Demux2/5 -> individual3/5(reg_in4)
  Demux2/4 -> individual3/4(reg_in3)
  Demux2/3 -> individual3/3(reg_in2)
  Demux2/2 -> individual3/2(reg_in1)
  Demux2/1 -> individual3/1(reg_in)
  Demux1/6 -> individual2/6(reg_in5)
  Demux1/5 -> individual2/5(reg_in4)
  Demux1/4 -> individual2/4(reg_in3)
  Demux1/3 -> individual2/3(reg_in2)
  Demux1/2 -> individual2/2(reg_in1)
  Demux1/1 -> individual2/1(reg_in)
  Demux1/7 -> individual2/7(reg_in6)
  individual2/7(b4) -> Mux2/7
  individual2/6(b3) -> Mux2/6
  individual2/5(b2) -> Mux2/5
  individual2/4(a4) -> Mux2/4
  individual1/7(b4) -> Mux1/7
  Demux/7 -> individual1/7(reg_in6)
  Mux4/1 -> output_selector/5(In5), Switch6/3
  Chart/2(index_reset) -> [index_reset]
  [index_reset] -> swap_counter1/2(In2)
  [index_increment] -> swap_counter1/1(In1)
  Constant14/1 -> Relational Operator14/2
  Relational Operator14/1 -> Logical Operator5/2
  Relational Operator13/1 -> Logical Operator4/2
  Constant7/1 -> Relational Operator13/2
  Relational Operator12/1 -> Logical Operator3/2
  Constant6/1 -> Relational Operator12/2
  Relational Operator11/1 -> Logical Operator2/2
  Constant5/1 -> Relational Operator11/2
  chose_output/1 -> [chose_out_port]
  Chart/3(sort_done) -> sort_done/1
  [start_sort] -> Chart/2(start_sort)
  individual2/3(a3) -> Mux2/3
  individual1/4(a4) -> Mux1/4
  Demux/4 -> individual1/4(reg_in3)
  individual1/2(a2) -> Mux1/2
  Relational Operator4/1 -> individual1/8(enable)
  individual1/6(b3) -> Mux1/6
  Demux/2 -> individual1/2(reg_in1)
  individual1/5(b2) -> Mux1/5
  Logical Operator2/1 -> Relational Operator4/1
  Constant10/1 -> Relational Operator7/2
  Relational Operator9/1 -> Logical Operator1/2
  Switch2/1 -> Demux/1
  Multiport Switch1/1 -> Relational Operator/2
  Relational Operator7/1 -> Switch6/2, Logical Operator1/1
  individual2/2(a2) -> Mux2/2
  Switch5/1 -> Demux2/1
  Chart/1(index_increment) -> [index_increment]
  Switch7/1 -> Demux3/1
  Constant8/1 -> Relational Operator5/2
  individual3/1(score) -> Multiport Switch/4, Multiport Switch1/3, Mux3/1
  Mux2/1 -> Switch6/1, Switch2/1, output_selector/3(In3)
  Demux/3 -> individual1/3(reg_in2)
  Logical Operator4/1 -> individual3/8(enable)
  Relational Operator/1 -> Chart/4(swap_signal)
  chose_input/1 -> Relational Operator11/1, Relational Operator12/1, Relational Operator13/1, Relational Operator14/1
  Demux/6 -> individual1/6(reg_in5)
  [chose_out_port] -> output_selector/1(chose_port)
  individual2/1(score) -> Multiport Switch1/2, Multiport Switch1/5, Multiport Switch/3, Mux2/1
  output_selector/1(Out1) -> individual_out/1
  Switch6/1 -> Switch5/1
  [commit_swap_index] -> Relational Operator10/1
  Constant12/1 -> Relational Operator9/2
  Constant13/1 -> Relational Operator10/2
  Constant4/1 -> Relational Operator4/2
  Relational Operator6/1 -> Switch4/2, Logical Operator/1
  individual4/1(score) -> Mux4/1, Multiport Switch1/4
  Switch3/1 -> Demux1/1
  individual_in/1 -> Switch2/3, Switch3/3, Switch5/3, Switch7/3
  Demux/5 -> individual1/5(reg_in4)
  Logical Operator/1 -> Switch3/2, Logical Operator3/1
  Chart/4(commit_swap) -> [commit_swap_index]
  start_sorting/1 -> [start_sort]
  Constant11/1 -> Relational Operator8/2
  Multiport Switch/1 -> Relational Operator/1
  Logical Operator5/1 -> individual4/8(enable)
  Logical Operator3/1 -> individual2/8(enable)
  [commit_swap_index] -> Relational Operator7/1, Relational Operator9/1
  [commit_swap_index] -> Relational Operator6/1, Relational Operator8/1
  Relational Operator8/1 -> Logical Operator/2
  Chart/6(reset_swaps) -> [reset_swaps]
  Mux1/1 -> elite_individual/1, output_selector/2(In2), Switch4/1
  [commit_swap_index] -> Relational Operator5/1
  [swaps_increment] -> swap_counter/1(In1)
  Relational Operator5/1 -> Switch2/2, Logical Operator2/1
  individual1/3(a3) -> Mux1/3
  swap_counter/1(Out1) -> Chart/3(swaps_in)
  [reset_swaps] -> swap_counter/2(In2)
  Relational Operator10/1 -> Switch7/2, Logical Operator5/1
  Mux3/1 -> Switch7/1, Switch4/3, output_selector/4(In4)
  Demux/1 -> individual1/1(reg_in)
  individual1/1(score) -> Multiport Switch/2, Multiport Switch/5, Mux1/1
  Switch4/1 -> Switch3/1
  swap_counter1/1(Out1) -> Chart/1(index), Multiport Switch/1, Multiport Switch1/1
  Chart/5(swaps_increment) -> [swaps_increment]
  Constant9/1 -> Relational Operator6/2
  Logical Operator1/1 -> Switch5/2, Logical Operator4/1

== system DUALportRAMinterface_v2/PL/integration_block1/GA_main/generation_counter ==
  In1 : Inport
  In2 : Inport  Port=2
  Add : Sum  OutDataTypeStr=fixdt(0,16,0)  AccumDataTypeStr=fixdt(0,16,0)
  Constant18 : Constant  OutDataTypeStr=fixdt(0,16,0)  SampleTime=Ts
  Constant19 : Constant  Value=0  OutDataTypeStr=fixdt(0,16,0)  SampleTime=Ts
  Constant20 : Constant  Value=0  OutDataTypeStr=fixdt(0,16,0)  SampleTime=Ts
  Delay : Delay  DelayLength=1  InitialCondition=0  SampleTime=Ts
  Switch : Switch  Criteria=u2 > Threshold  OutDataTypeStr=fixdt(0,16,0)  SaturateOnIntegerOverflow=off  InputSameDT=off
  Switch8 : Switch  Criteria=u2 > Threshold  OutDataTypeStr=fixdt(0,16,0)  SaturateOnIntegerOverflow=off  InputSameDT=off
  Out1 : Outport
  wires:
  Constant19/1 -> Switch/3
  Switch8/1 -> Add/2
  Switch/1 -> Add/1
  Delay/1 -> Out1/1, Switch8/3
  In2/1 -> Switch8/2
  Add/1 -> Delay/1
  Constant20/1 -> Switch8/1
  Constant18/1 -> Switch/1
  In1/1 -> Switch/2

== system DUALportRAMinterface_v2/PL/integration_block1/GA_main/index_counter ==
  In1 : Inport
  In2 : Inport  Port=2
  Add : Sum  OutDataTypeStr=fixdt(0,4,0)  AccumDataTypeStr=fixdt(0,4,0)
  Constant18 : Constant  OutDataTypeStr=fixdt(0,4,0)  SampleTime=Ts
  Constant19 : Constant  Value=0  OutDataTypeStr=fixdt(0,4,0)  SampleTime=Ts
  Constant20 : Constant  Value=0  OutDataTypeStr=fixdt(0,4,0)  SampleTime=Ts
  Delay : Delay  DelayLength=1  InitialCondition=0  SampleTime=Ts
  Switch : Switch  Criteria=u2 > Threshold  OutDataTypeStr=fixdt(0,4,0)  SaturateOnIntegerOverflow=off  InputSameDT=off
  Switch8 : Switch  Criteria=u2 > Threshold  OutDataTypeStr=fixdt(0,4,0)  SaturateOnIntegerOverflow=off  InputSameDT=off
  index_counter : Outport
  wires:
  Constant19/1 -> Switch/3
  Switch8/1 -> Add/2
  Switch/1 -> Add/1
  Delay/1 -> index_counter/1, Switch8/3
  In2/1 -> Switch8/2
  Add/1 -> Delay/1
  Constant20/1 -> Switch8/1
  Constant18/1 -> Switch/1
  In1/1 -> Switch/2

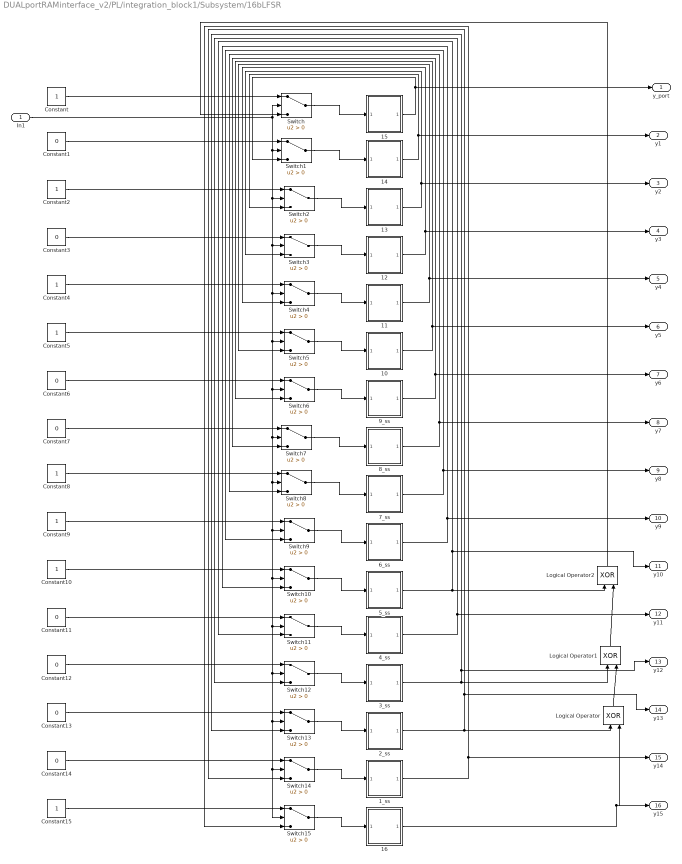
== system DUALportRAMinterface_v2/PL/integration_block1/Subsystem/16bLFSR ==
  In1 : Inport
  10 : Subsystem
  11 : Subsystem
  12 : Subsystem
  13 : Subsystem
  14 : Subsystem
  15 : Subsystem
  16 : Subsystem
  1_ss : Subsystem
  2_ss : Subsystem
  3_ss : Subsystem
  4_ss : Subsystem
  5_ss : Subsystem
  6_ss : Subsystem
  7_ss : Subsystem
  8_ss : Subsystem
  9_ss : Subsystem
  Constant{,2,4..5,8..10,15} (8 alike) : Constant  OutDataTypeStr=boolean  SampleTime=Ts
  Constant{1,3,6..7,11..14} (8 alike) : Constant  Value=0  OutDataTypeStr=boolean  SampleTime=Ts
  Logical Operator : Logic  Operator=XOR  IconShape=distinctive  AllPortsSameDT=off  OutDataTypeStr=boolean
  Logical Operator1 : Logic  Operator=XOR  IconShape=distinctive  AllPortsSameDT=off  OutDataTypeStr=boolean
  Logical Operator2 : Logic  Operator=XOR  IconShape=distinctive  AllPortsSameDT=off  OutDataTypeStr=boolean
  Switch{,1..15} (16 alike) : Switch  Criteria=u2 > Threshold  SaturateOnIntegerOverflow=off  InputSameDT=off
  y_port : Outport
  y1 : Outport  Port=2
  y2 : Outport  Port=3
  y3 : Outport  Port=4
  y4 : Outport  Port=5
  y5 : Outport  Port=6
  y6 : Outport  Port=7
  y7 : Outport  Port=8
  y8 : Outport  Port=9
  y9 : Outport  Port=10
  y10 : Outport  Port=11
  y11 : Outport  Port=12
  y12 : Outport  Port=13
  y13 : Outport  Port=14
  y14 : Outport  Port=15
  y15 : Outport  Port=16
  wires:
  5_ss/1(reg_out) -> Logical Operator2/1, y10/1, Switch11/3
  6_ss/1(reg_out) -> y9/1, Switch10/3
  2_ss/1(reg_out) -> Logical Operator/1, y13/1, Switch14/3
  11/1(reg_out) -> y4/1, Switch5/3
  Logical Operator2/1 -> Switch/3
  Constant13/1 -> Switch13/1
  Switch13/1 -> 2_ss/1(reg_in)
  3_ss/1(reg_out) -> Logical Operator1/1, y12/1, Switch13/3
  4_ss/1(reg_out) -> y11/1, Switch12/3
  Constant/1 -> Switch/1
  Constant4/1 -> Switch4/1
  Constant2/1 -> Switch2/1
  In1/1 -> Switch/2, Switch15/2, Switch14/2, Switch13/2, Switch12/2, Switch11/2, Switch10/2, Switch9/2, Switch8/2, Switch7/2, Switch6/2, Switch5/2, Switch4/2, Switch3/2, Switch2/2, Switch1/2
  Switch12/1 -> 3_ss/1(reg_in)
  15/1(reg_out) -> y_port/1, Switch1/3
  Switch1/1 -> 14/1(reg_in)
  Constant8/1 -> Switch8/1
  Constant6/1 -> Switch6/1
  Constant5/1 -> Switch5/1
  Constant14/1 -> Switch14/1
  Constant11/1 -> Switch11/1
  Switch5/1 -> 10/1(reg_in)
  Constant9/1 -> Switch9/1
  Logical Operator/1 -> Logical Operator1/2
  Switch2/1 -> 13/1(reg_in)
  7_ss/1(reg_out) -> y8/1, Switch9/3
  Logical Operator1/1 -> Logical Operator2/2
  Switch11/1 -> 4_ss/1(reg_in)
  Constant7/1 -> Switch7/1
  Switch6/1 -> 9_ss/1(reg_in)
  Switch/1 -> 15/1(reg_in)
  Constant12/1 -> Switch12/1
  Switch4/1 -> 11/1(reg_in)
  Constant15/1 -> Switch15/1
  16/1(reg_out) -> y15/1, Logical Operator/2
  13/1(reg_out) -> y2/1, Switch3/3
  Switch9/1 -> 6_ss/1(reg_in)
  Switch7/1 -> 8_ss/1(reg_in)
  Constant10/1 -> Switch10/1
  Switch14/1 -> 1_ss/1(reg_in)
  Switch3/1 -> 12/1(reg_in)
  Switch15/1 -> 16/1(reg_in)
  9_ss/1(reg_out) -> y6/1, Switch7/3
  Constant3/1 -> Switch3/1
  Constant1/1 -> Switch1/1
  14/1(reg_out) -> y1/1, Switch2/3
  Switch10/1 -> 5_ss/1(reg_in)
  10/1(reg_out) -> y5/1, Switch6/3
  Switch8/1 -> 7_ss/1(reg_in)
  12/1(reg_out) -> y3/1, Switch4/3
  8_ss/1(reg_out) -> y7/1, Switch8/3
  1_ss/1(reg_out) -> y14/1, Switch15/3

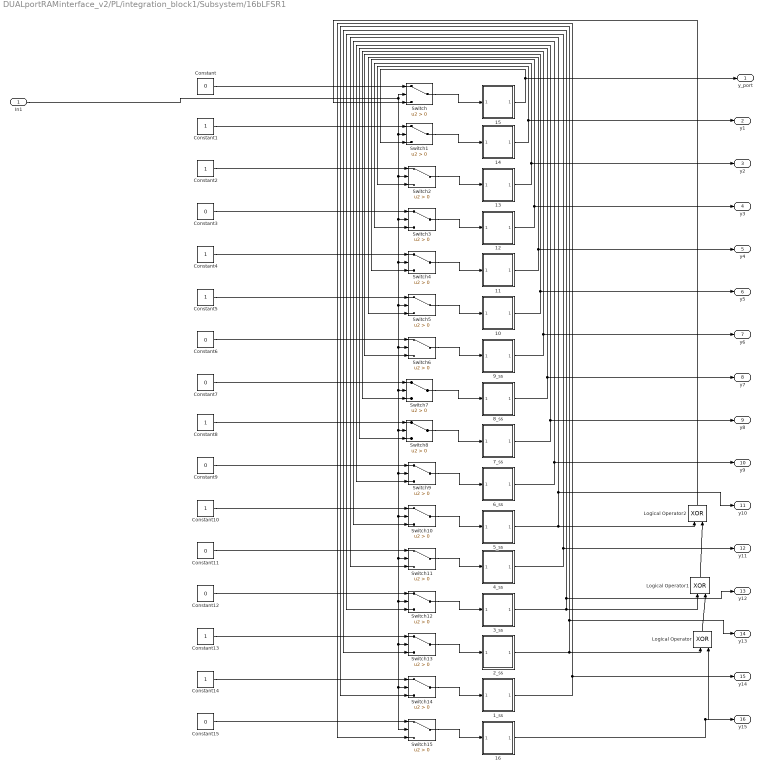
== system DUALportRAMinterface_v2/PL/integration_block1/Subsystem/16bLFSR1 ==
  In1 : Inport
  10 : Subsystem
  11 : Subsystem
  12 : Subsystem
  13 : Subsystem
  14 : Subsystem
  15 : Subsystem
  16 : Subsystem
  1_ss : Subsystem
  2_ss : Subsystem
  3_ss : Subsystem
  4_ss : Subsystem
  5_ss : Subsystem
  6_ss : Subsystem
  7_ss : Subsystem
  8_ss : Subsystem
  9_ss : Subsystem
  Constant{,3,6..7,9,11..12,15} (8 alike) : Constant  Value=0  OutDataTypeStr=boolean  SampleTime=Ts
  Constant{1..2,4..5,8,10,13..14} (8 alike) : Constant  OutDataTypeStr=boolean  SampleTime=Ts
  Logical Operator : Logic  Operator=XOR  IconShape=distinctive  AllPortsSameDT=off  OutDataTypeStr=boolean
  Logical Operator1 : Logic  Operator=XOR  IconShape=distinctive  AllPortsSameDT=off  OutDataTypeStr=boolean
  Logical Operator2 : Logic  Operator=XOR  IconShape=distinctive  AllPortsSameDT=off  OutDataTypeStr=boolean
  Switch{,1..15} (16 alike) : Switch  Criteria=u2 > Threshold  SaturateOnIntegerOverflow=off  InputSameDT=off
  y_port : Outport
  y1 : Outport  Port=2
  y2 : Outport  Port=3
  y3 : Outport  Port=4
  y4 : Outport  Port=5
  y5 : Outport  Port=6
  y6 : Outport  Port=7
  y7 : Outport  Port=8
  y8 : Outport  Port=9
  y9 : Outport  Port=10
  y10 : Outport  Port=11
  y11 : Outport  Port=12
  y12 : Outport  Port=13
  y13 : Outport  Port=14
  y14 : Outport  Port=15
  y15 : Outport  Port=16
  wires:
  1_ss/1(reg_out) -> Switch15/3, y14/1
  8_ss/1(reg_out) -> Switch8/3, y7/1
  12/1(reg_out) -> Switch4/3, y3/1
  Switch8/1 -> 7_ss/1(reg_in)
  10/1(reg_out) -> Switch6/3, y5/1
  Switch10/1 -> 5_ss/1(reg_in)
  14/1(reg_out) -> Switch2/3, y1/1
  Constant1/1 -> Switch1/1
  Constant3/1 -> Switch3/1
  9_ss/1(reg_out) -> Switch7/3, y6/1
  Switch15/1 -> 16/1(reg_in)
  Switch3/1 -> 12/1(reg_in)
  Switch14/1 -> 1_ss/1(reg_in)
  Constant10/1 -> Switch10/1
  Switch7/1 -> 8_ss/1(reg_in)
  Switch9/1 -> 6_ss/1(reg_in)
  13/1(reg_out) -> Switch3/3, y2/1
  16/1(reg_out) -> Logical Operator/2, y15/1
  Constant15/1 -> Switch15/1
  Switch4/1 -> 11/1(reg_in)
  Constant12/1 -> Switch12/1
  Switch/1 -> 15/1(reg_in)
  Switch6/1 -> 9_ss/1(reg_in)
  Constant7/1 -> Switch7/1
  Switch11/1 -> 4_ss/1(reg_in)
  Logical Operator1/1 -> Logical Operator2/2
  7_ss/1(reg_out) -> Switch9/3, y8/1
  Switch2/1 -> 13/1(reg_in)
  Logical Operator/1 -> Logical Operator1/2
  Constant9/1 -> Switch9/1
  Switch5/1 -> 10/1(reg_in)
  Constant11/1 -> Switch11/1
  Constant14/1 -> Switch14/1
  Constant5/1 -> Switch5/1
  Constant6/1 -> Switch6/1
  Constant8/1 -> Switch8/1
  Switch1/1 -> 14/1(reg_in)
  15/1(reg_out) -> Switch1/3, y_port/1
  Switch12/1 -> 3_ss/1(reg_in)
  In1/1 -> Switch1/2, Switch2/2, Switch3/2, Switch4/2, Switch5/2, Switch6/2, Switch7/2, Switch8/2, Switch9/2, Switch10/2, Switch11/2, Switch12/2, Switch13/2, Switch14/2, Switch15/2, Switch/2
  Constant2/1 -> Switch2/1
  Constant4/1 -> Switch4/1
  Constant/1 -> Switch/1
  4_ss/1(reg_out) -> Switch12/3, y11/1
  3_ss/1(reg_out) -> Switch13/3, y12/1, Logical Operator1/1
  Switch13/1 -> 2_ss/1(reg_in)
  Constant13/1 -> Switch13/1
  Logical Operator2/1 -> Switch/3
  11/1(reg_out) -> Switch5/3, y4/1
  2_ss/1(reg_out) -> Switch14/3, y13/1, Logical Operator/1
  6_ss/1(reg_out) -> Switch10/3, y9/1
  5_ss/1(reg_out) -> Switch11/3, y10/1, Logical Operator2/1
